simulink model "PV_model_final_02"  (R2021b)
settings: Solver=FixedStepDiscrete  StartTime=0.0  StopTime=80  FixedStep=Ts_Power  RelTol=1e-3
InitFcn:
  | freq = 60;
  | n = 100;
  | a = 20;
  | b = 10;
  | c = 150;
  | 
  | Fc = n * freq; % Carrier frequency, used for generating inverter SPWM signal (Hz)
  | Ts_Power = 1/(a * Fc); % SPS sample time (sec)
  | Ts_Control = b * Ts_Power; % Inverter control sample time (sec)
  | Ts_Data = c * Ts_Power; % Data storage and scope sample time (sec)
  | 
  | Dbias = 0.0;
  | Dupperlim = 0.5;
  | Dlowerlim = 0.2;
  | 
  | Ron=75e-3;
StopFcn:
  | %load('temp1.mat')
  | %[c,hist,edges,rmm,idx] = rainflow(temp.Data(:,3),temp.Time);
  | %histogram('BinEdges',edges','BinCounts',sum(hist,2));
  | %title('Histogram of S5 Thermal Cycles')
  | %xlabel('Temperature Cycle Range')
  | %ylabel('Cycle count')
undefined symbols (not defined in the file or in its folder): DiscIntNeverNeededParam
libraries: spsParallelRLCBranchLib x11, spsSeriesRLCBranchLib x6, spsMeanLib x6, spsIGBTDiodeLib x4, spsTHDLib x4, spsVoltageMeasurementLib x3, spsCurrentMeasurementLib x2, spsDiodeLib x2, spsGroundLib x2, slpidlib x2, spsControlledCurrentSourceLib x2, spsACVoltageSourceLib x1
settings Model: SimulationMode=accelerator  Creator=niall  LastModifiedBy=niall
settings DataIOCC: SaveOutput=off  DSMLogging=off  SaveTime=off  ReturnWorkspaceOutputs=off  SignalLoggingName=simout  LoggingToFile=on  LoggingFileName=simout.mat
settings DebuggingCC: ReadBeforeWriteMsg=DisableAll  WriteAfterWriteMsg=DisableAll  WriteAfterReadMsg=DisableAll  MultiTaskDSMMsg=none
settings ModelReferenceCC: UpdateModelReferenceTargets=IfOutOfDate
settings SFSimCC: SFSimEcho=off

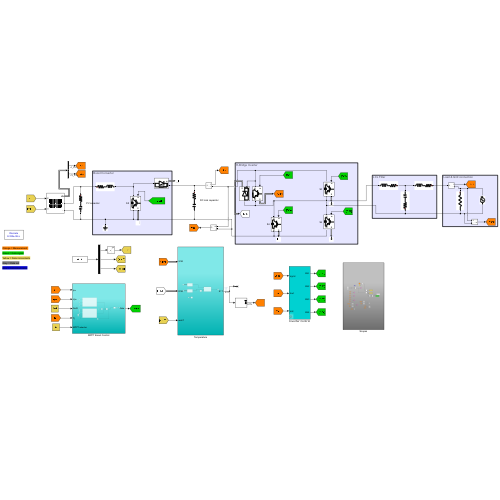
[thumbnail: Simulink's stored preview of the top-level diagram]
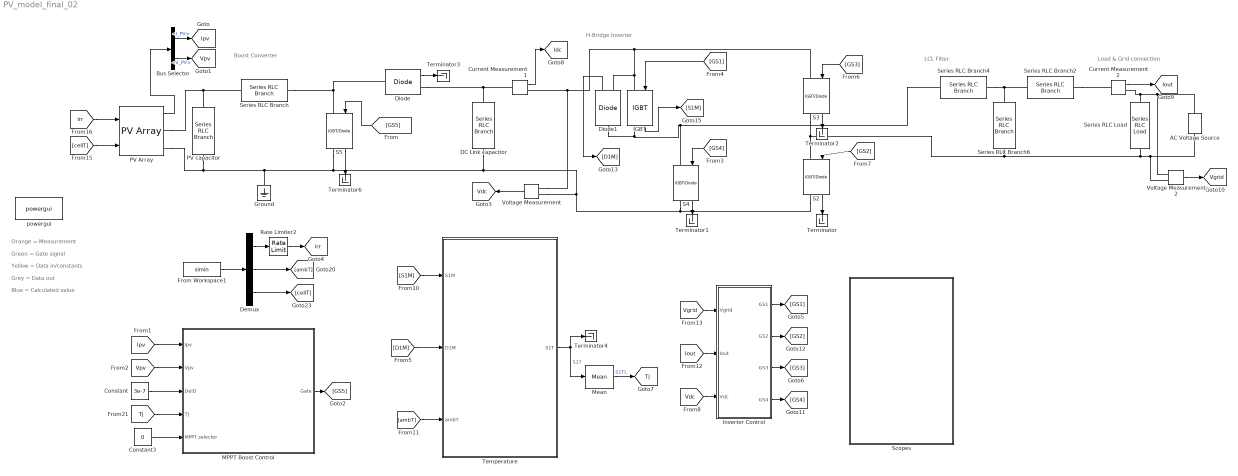
== system PV_model_final_02 ==
  note: Blue = Calculated value
  note: Grey = Data out
  note: Boost Converter
  note: H-Bridge Inverter
  note: LCL Filter
  note: Yellow = Data in/constants
  note: Green = Gate signal
  note: Orange = Measurement
  note: Load & Grid connection
  AC Voltage Source : spsACVoltageSourceLib/AC Voltage Source  Amplitude=240*sqrt(2)  Phase=0  Frequency=60  SampleTime=Ts_Power  Measurements=None  BusType=swing  Pref=10e3  Qref=0  Qmin=-inf  Qmax=+inf
  Bus Selector : BusSelector  OutputSignals=I_PV,V_PV
  Constant : Constant  Value=3e-7
  Constant3 : Constant  Value=0
  Current Measurement1 : spsCurrentMeasurementLib/Current Measurement  PhasorSimulation=off  OutputType=Complex  PSBequivalent=0
  Current Measurement2 : spsCurrentMeasurementLib/Current Measurement  PhasorSimulation=off  OutputType=Complex  PSBequivalent=0
  DC Link capacitor : spsSeriesRLCBranchLib/Series RLC Branch  LConnTagsString=__new0  RConnTagsString=__new0  BranchType=RC  Resistance=2.2e-3  Inductance=1e-3  SetiL0=off  InitialCurrent=0  Capacitance=2100e-6  Setx0=on  InitialVoltage=450  Measurements=None
  Demux : Demux  Outputs=3
  Diode : spsDiodeLib/Diode  Ron=0.001  Lon=0  Vf=0.8  IC=0  UseSnubber=0  Rs=500  Cs=250e-9  Measurements=on
  Diode1 : spsDiodeLib/Diode  Ron=10e-3  Lon=0  Vf=0.8  IC=0  UseSnubber=0  Rs=500  Cs=250e-9  Measurements=on
  From Workspace1 : FromWorkspace  VariableName=simin  SampleTime=Ts_Power  OutputAfterFinalValue=Holding final value
  Ground : spsGroundLib/Ground  LConnTagsString=a
  IGBT : spsIGBTLib/IGBT  Ron=Ron  Lon=0  Vf=2.2  Tf=1e-6  Tt=2e-6  IC=0  Rs=1e5  Cs=inf  Measurements=on
  Inverter Control : Subsystem  mask(Inverter Control){Pnom=10000, Fnom=60, Vnom_prim=240, Vnom_dc=450, Kp_VDCreg=10, Ki_VDCreg=50, Kp_Ireg=0.3, Ki_Ireg=9, RLff=[ 0.004 0.2 ], Fc=Fc, PWMmode12=Bipolar, Ts_Control=Ts_Control, Ts_PWMgenerator=Ts_Power}
      mask prompts: Pnom "Power (VA)"; Fnom "Frequency (Hz)"; Vnom_prim "Primary voltage (Vrms LL)"; Vnom_dc "DC voltage (V)"; Kp_VDCreg "Proportional gain"; Ki_VDCreg "Integral gain"; Kp_Ireg "Proportional gain"; Ki_Ireg "Integral gain"; RLff "Feedforward Values [Rff Lff] (pu)"; Fc "Carrier frequency (Hz)"; PWMmode12 "PWM method"; Ts_Control "Control systems"; Ts_PWMgenerator "PWM generator"
      mask help:
      | The main components of the Inverter Control are:
      | 1. PLL & Measurements
      | 2. Maximum Power Point Tracker System (MPPT) using a Perturb & Observe algorithm
      | 3. DC Voltage Regulator
      | 4. Current Regulator
      | 5. PWM Modulator
      mask init:
      | blockName=gcb;
      | if PWMmode12==1
      |     set_param([blockName,'/','PWM_Generator'],'ModulatorType','Single-phase full-bridge (4 pulses)')
      | else
      |     set_param([blockName,'/','PWM_Generator'],'ModulatorType','Single-phase full-bridge - Bipolar modulation (4 pulses)')
      | end
      mask TypeOptions PWMmode12: Unipolar | Bipolar
      mask DialogControl Container4 Prompt: Nominal Values:
      mask DialogControl Container8 Prompt: Dc Voltage Regulator:
      mask DialogControl Container6 Prompt: Current Regulator:
      mask DialogControl Container9 Prompt: PWM Modulator:
      mask DialogControl SampleTimes Prompt: Sample Times:
  MPPT Boost Control : Subsystem
  Mean : spsMeanLib/Mean  Freq=1  Vinit=20  Ts=Ts_Power
  PV Array : spsPVArrayLib/PV Array  Npar=2  Nser=9  PlotType=array @ 1000 W/m2 & specified temperatures  S_vec="[ 1000  500  100 ]"  Temp_C_vec="[ 45 25  ]"  ModuleName=User-defined  PlotWhenSelected=off  Pm=554.91  Ncell=110  Voc=38.1  Isc=18.56  Vm=31.8  Im=17.45  beta_Voc_pc=-0.25  alpha_Isc_pc=0.04  beta_Voc=-0.09525  alpha_Isc=0.007424  IL=18.6423  I0=6.4129e-12  nI=0.4702  Rsh=76.5819  Rs=0.11972  RobustModel=off  RobustCellTemperature=313.3991  BAL=on  Tc=1e-6  Tfilter=5e-5
  PV capacitor : spsSeriesRLCBranchLib/Series RLC Branch  LConnTagsString=__new0  RConnTagsString=__new0  BranchType=RC  Resistance=2.2e-3  Inductance=1e-3  SetiL0=off  InitialCurrent=0  Capacitance=2100e-6  Setx0=off  InitialVoltage=0  Measurements=None
  Rate Limiter2 : RateLimiter  RisingSlewLimit=2000  FallingSlewLimit=-2000  SampleTimeMode=inherited
  S{2..5} (4 alike) : spsIGBTDiodeLib/IGBT//Diode  Ron=Ron  Rs=1e5  Cs=inf  Measurements=on
  Scopes : Subsystem
  Series RLC Branch : spsSeriesRLCBranchLib/Series RLC Branch  LConnTagsString=__new0  RConnTagsString=__new0  BranchType=RL  Resistance=2e-3  Inductance=1.5e-3  SetiL0=off  InitialCurrent=0  Capacitance=1e-6  Setx0=off  InitialVoltage=0  Measurements=None
  Series RLC Branch2 : spsSeriesRLCBranchLib/Series RLC Branch  LConnTagsString=__new0  RConnTagsString=__new0  BranchType=RL  Resistance=4e-3  Inductance=4e-3  SetiL0=off  InitialCurrent=0  Capacitance=1e-6  Setx0=off  InitialVoltage=0  Measurements=None
  Series RLC Branch4 : spsSeriesRLCBranchLib/Series RLC Branch  LConnTagsString=__new0  RConnTagsString=__new0  BranchType=RL  Resistance=4e-3  Inductance=8e-3  SetiL0=off  InitialCurrent=0  Capacitance=1e-6  Setx0=off  InitialVoltage=0  Measurements=None
  Series RLC Branch6 : spsSeriesRLCBranchLib/Series RLC Branch  LConnTagsString=__new0  RConnTagsString=__new0  BranchType=RC  Resistance=2e-3  Inductance=1e-3  SetiL0=off  InitialCurrent=0  Capacitance=5e-6  Setx0=off  InitialVoltage=0  Measurements=None
  Series RLC Load : spsSeriesRLCLoadLib/Series RLC Load  LConnTagsString=a  RConnTagsString=__new0  NominalVoltage=240  NominalFrequency=60  ActivePower=10e3  InductivePower=0  CapacitivePower=0  Setx0=off  InitialVoltage=0  SetiL0=off  InitialCurrent=0  Measurements=None  LoadType=constant Z
  Temperature : Subsystem
  Terminator{,1..4,6} (6 alike) : Terminator
  Voltage Measurement : spsVoltageMeasurementLib/Voltage Measurement  PhasorSimulation=off  OutputType=Complex  PSBequivalent=0
  Voltage Measurement2 : spsVoltageMeasurementLib/Voltage Measurement  PhasorSimulation=off  OutputType=Complex  PSBequivalent=0
  powergui : spspowerguiLib/powergui  Priority=1  SimulationMode=Discrete  SampleTime=Ts_Power  frequency=60  Iterations=50  frequencyindice=0  Pbase=100e6  ErrMax=1e-4  UnitsV=kV  UnitsW=MW  buscounter=0  FunctionMessages=off  echomessages=off  EnableUseOfTLC=off  CurrentSourceSwitches=off  DisableSnubberDevices=off  DisableRonSwitches=off  DisableVfSwitches=off  DisplayEquations=off  AutomaticDiscreteSolvers=off  SolverType=Tustin/Backward Euler (TBE)  Interpol=off  ExternalGateDelay=off  methode=off  Ts=100  x0status=blocks  SPID=on  SwTol=0  HookPort=off  NonlinearTolerance=1e-4  nMaxIteration=100  ContinueOnMaxIteration=off  RestoreLinks=warning  ResistiveCurrentMeasurement=off  Frange=[0:2:500]  Ylog=off  Xlog=on  ShowGrid=off  save=off  variable=ZData  structure=0  ZoomFFT=off  StartTime=0.0  cycles=1  DisplayStyle=1  fundamental=60  FreqAxis=off  MaxFrequency=1000  frequencyindicesteady=1  RmsSteady=1  display=off
  tag scope: Idc=global, Iout=global, Ipv=global, Tj=global, Vdc=global, Vgrid=global, Vpv=global, irr=global
  wires:
  MPPT Boost Control/1(Gate) -> [GS5]
  [GS5] -> S5/1
  Current Measurement1/1 -> [Idc]
  [cellT] -> PV Array/2
  Bus Selector/2 -> [Vpv]  "<V_PV>"
  Voltage Measurement/1 -> [Vdc]
  Bus Selector/1 -> [Ipv]  "<I_PV>"
  [Ipv] -> MPPT Boost Control/1(Ipv)
  [Vpv] -> MPPT Boost Control/2(Vpv)
  Constant/1 -> MPPT Boost Control/3(DelD)
  PV Array/1 -> Bus Selector/1
  Current Measurement2/1 -> [Iout]
  Voltage Measurement2/1 -> [Vgrid]
  [Vdc] -> Inverter Control/3(Vdc)
  [Iout] -> Inverter Control/2(Iout)
  [Vgrid] -> Inverter Control/1(Vgrid)
  [GS1] -> IGBT/1
  [GS3] -> S3/1
  [GS4] -> S4/1
  [GS2] -> S2/1
  IGBT/1 -> [S1M]
  [S1M] -> Temperature/1(S1M)
  [ambT] -> Temperature/3(ambT)
  Inverter Control/1(GS1) -> [GS1]
  Inverter Control/2(GS2) -> [GS2]
  Inverter Control/3(GS3) -> [GS3]
  Inverter Control/4(GS4) -> [GS4]
  Temperature/1(S1T) -> Terminator4/1, Mean/1  "S1T"
  [Tj] -> MPPT Boost Control/4(Tj)
  Constant3/1 -> MPPT Boost Control/5(MPPT selector)
  Demux/1 -> Rate Limiter2/1
  From Workspace1/1 -> Demux/1
  Demux/2 -> [ambT]
  Demux/3 -> [cellT]
  S2/1 -> Terminator/1
  S4/1 -> Terminator1/1
  S3/1 -> Terminator2/1
  Diode/1 -> Terminator3/1
  Mean/1 -> [Tj]  "S1TL"
  [irr] -> PV Array/1
  Rate Limiter2/1 -> [irr]
  S5/1 -> Terminator6/1
  Diode1/1 -> [D1M]
  [D1M] -> Temperature/2(D1M)
  connections:
  DC Link capacitor/LConn1 -- Diode/RConn1 -- Current Measurement1/LConn1
  DC Link capacitor/RConn1 -- S5/RConn1 -- PV Array/RConn2 -- PV capacitor/RConn1 -- Ground/LConn1 -- S2/RConn1 -- S4/RConn1 -- Voltage Measurement/LConn2
  PV Array/RConn1 -- Series RLC Branch/LConn1 -- PV capacitor/LConn1
  S4/LConn1 -- Diode1/LConn1 -- IGBT/RConn1 -- Series RLC Branch4/RConn1
  AC Voltage Source/RConn1 -- Current Measurement2/RConn1 -- Series RLC Load/LConn1 -- Voltage Measurement2/LConn1
  Series RLC Branch4/LConn1 -- Series RLC Branch6/RConn1 -- Series RLC Branch2/RConn1
  Series RLC Branch/RConn1 -- S5/LConn1 -- Diode/LConn1
  Series RLC Load/RConn1 -- AC Voltage Source/LConn1 -- Voltage Measurement2/LConn2 -- S3/RConn1 -- S2/LConn1 -- Series RLC Branch6/LConn1
  Series RLC Branch2/LConn1 -- Current Measurement2/LConn1
  Voltage Measurement/LConn1 -- S3/LConn1 -- Diode1/RConn1 -- IGBT/LConn1 -- Current Measurement1/RConn1

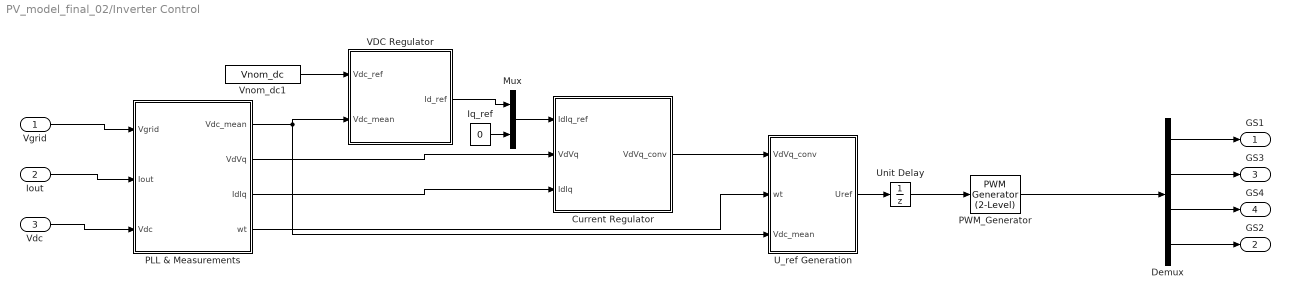
== system PV_model_final_02/Inverter Control ==
  Vgrid : Inport  PortDimensions=1
  Iout : Inport  Port=2  PortDimensions=1
  Vdc : Inport  Port=3  PortDimensions=1
  Current Regulator : Subsystem
  Demux : Demux
  Iq_ref : Constant  Value=0  SampleTime=Ts_Control
  Mux : Mux  Inputs=2
  PLL & Measurements : Subsystem
  PWM_Generator : spsPWMGenerator2LevelLib/PWM Generator (2-Level)  ModulatorType=Single-phase full-bridge - Bipolar modulation (4 pulses)  ModulatorMode=Unsynchronized  Fc=Fc  Pc=90  nF=27  MinMax="[ -1  1 ]"  SamplingTechnique=Asymmetrical regular (double edge)  ModulatingSignals=off  m=0.8  Freq=60  Phase=0  Ts=Ts_PWMgenerator  ShowCarrierOutport=off
      settings: AttributesFormatString=%<ModulatorType>
  "U_ref Generation " : Subsystem
  Unit Delay : UnitDelay  SampleTime=Ts_Control  HasFrameUpgradeWarning=on
  VDC Regulator : Subsystem
  Vnom_dc1 : Constant  Value=Vnom_dc  SampleTime=Ts_Control
  GS1 : Outport  VectorParamsAs1DForOutWhenUnconnected=off
  GS2 : Outport  Port=2  VectorParamsAs1DForOutWhenUnconnected=off
  GS3 : Outport  Port=3  VectorParamsAs1DForOutWhenUnconnected=off
  GS4 : Outport  Port=4  VectorParamsAs1DForOutWhenUnconnected=off
  wires:
  Iq_ref/1 -> Mux/2
  Vgrid/1 -> PLL & Measurements/1(Vgrid)
  Iout/1 -> PLL & Measurements/2(Iout)
  Unit Delay/1 -> PWM_Generator/1
  Vdc/1 -> PLL & Measurements/3(Vdc)
  PLL & Measurements/2(VdVq) -> Current Regulator/2(VdVq)
  PLL & Measurements/3(IdIq) -> Current Regulator/3(IdIq)
  Mux/1 -> Current Regulator/1(IdIq_ref)
  VDC Regulator/1(Id_ref) -> Mux/1
  PLL & Measurements/1(Vdc_mean) -> VDC Regulator/2(Vdc_mean), "U_ref Generation "/3(Vdc_mean)
  Current Regulator/1(VdVq_conv) -> "U_ref Generation "/1(VdVq_conv)
  PLL & Measurements/4(wt) -> "U_ref Generation "/2(wt)
  "U_ref Generation "/1(Uref) -> Unit Delay/1
  PWM_Generator/1 -> Demux/1
  Vnom_dc1/1 -> VDC Regulator/1(Vdc_ref)
  Demux/1 -> GS1/1
  Demux/2 -> GS3/1
  Demux/3 -> GS4/1
  Demux/4 -> GS2/1

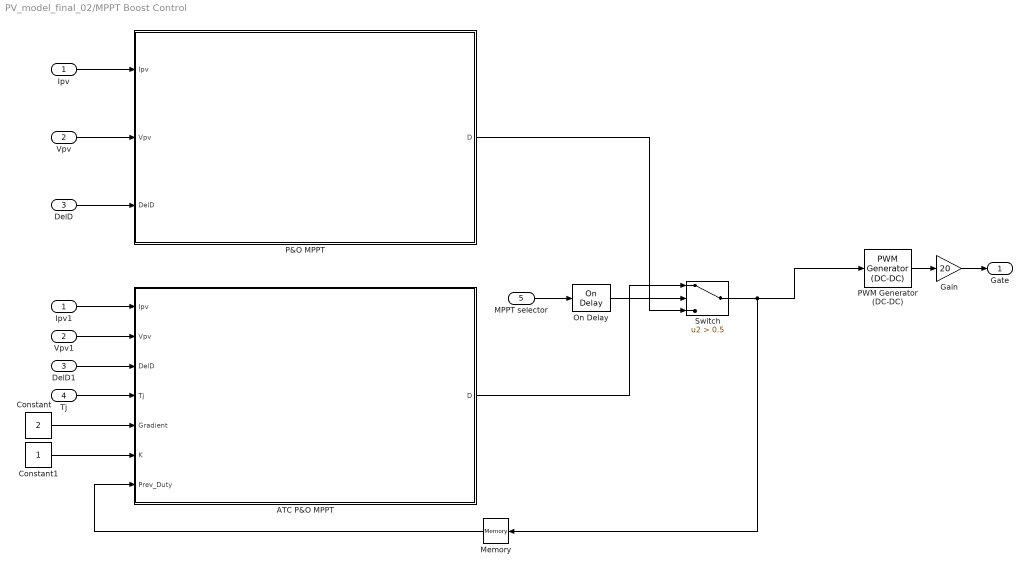
== system PV_model_final_02/MPPT Boost Control ==
  Ipv : Inport
  Vpv : Inport  Port=2
  DelD : Inport  Port=3
  Tj : Inport  Port=4
  MPPT selector : Inport  Port=5
  ATC P&O MPPT : Subsystem
  Constant : Constant  Value=2
  Constant1 : Constant
  DelD1 : InportShadow  Port=3
  Gain : Gain  Gain=20
  Ipv1 : InportShadow
  Memory : Memory
  On Delay : spsOnDelayLib/On Delay  DelayType=On delay  delay=5  ic=0  Ts=Ts_Control
      settings: SourceProductBaseCode=PS
  P&O MPPT : Subsystem
  PWM Generator (DC-DC) : spsPWMGeneratorDCDCLib/PWM Generator (DC-DC)  Fsw=5000  Ts=Ts_Power
  Switch : Switch  Criteria=u2 > Threshold  Threshold=0.5
  Vpv1 : InportShadow  Port=2
  Gate : Outport
  wires:
  Vpv/1 -> P&O MPPT/2(Vpv)
  Tj/1 -> ATC P&O MPPT/4(Tj)
  DelD/1 -> P&O MPPT/3(DelD)
  Ipv/1 -> P&O MPPT/1(Ipv)
  P&O MPPT/1(D) -> Switch/3
  DelD1/1 -> ATC P&O MPPT/3(DelD)
  Vpv1/1 -> ATC P&O MPPT/2(Vpv)
  Ipv1/1 -> ATC P&O MPPT/1(Ipv)
  ATC P&O MPPT/1(D) -> Switch/1
  MPPT selector/1 -> On Delay/1
  Constant/1 -> ATC P&O MPPT/5(Gradient)
  PWM Generator (DC-DC)/1 -> Gain/1
  Gain/1 -> Gate/1
  On Delay/1 -> Switch/2
  Memory/1 -> ATC P&O MPPT/7(Prev_Duty)
  Switch/1 -> PWM Generator (DC-DC)/1, Memory/1
  Constant1/1 -> ATC P&O MPPT/6(K)

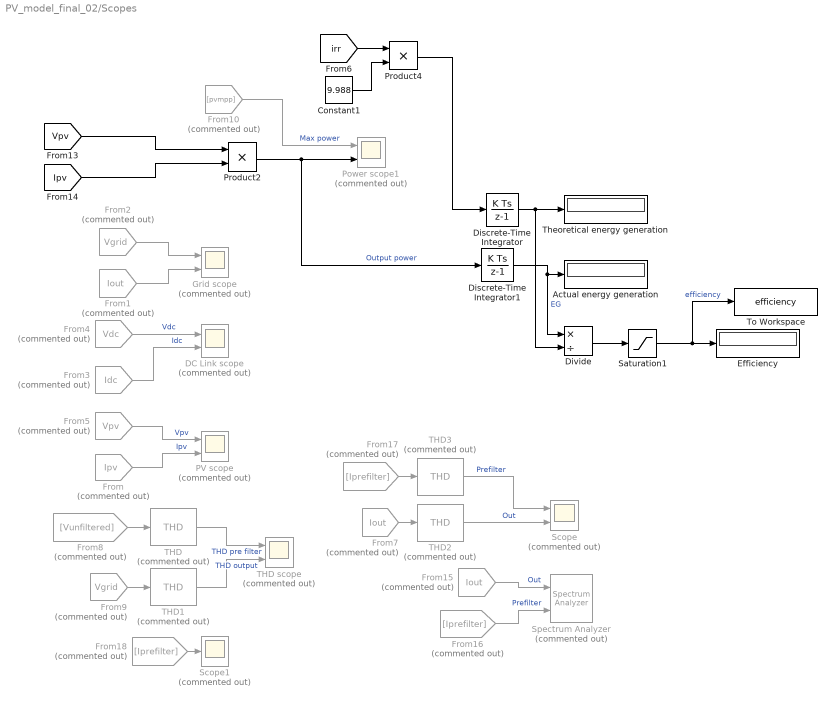
== system PV_model_final_02/Scopes ==
  Actual energy generation : Display
  Constant1 : Constant  Value=9.988  SampleTime=Ts_Power
  DC Link scope : Scope  Commented=on  NumInputPorts=2
  Discrete-Time Integrator : DiscreteIntegrator  SampleTime=Ts_Power  ICPrevOutput=DiscIntNeverNeededParam  ICPrevScaledInput=DiscIntNeverNeededParam
  Discrete-Time Integrator1 : DiscreteIntegrator  SampleTime=Ts_Power  ICPrevOutput=DiscIntNeverNeededParam  ICPrevScaledInput=DiscIntNeverNeededParam
  Divide : Product  Inputs=*/
  Efficiency : Display
  From : From  Commented=on  GotoTag=Ipv  TagVisibility=global
  From1 : From  Commented=on  GotoTag=Iout  TagVisibility=global
  From10 : From  Commented=on  GotoTag=pvmpp  TagVisibility=global
  From15 : From  Commented=on  GotoTag=Iout  TagVisibility=global
  From16 : From  Commented=on  GotoTag=Iprefilter  TagVisibility=global
  From17 : From  Commented=on  GotoTag=Iprefilter  TagVisibility=global
  From18 : From  Commented=on  GotoTag=Iprefilter  TagVisibility=global
  From2 : From  Commented=on  GotoTag=Vgrid  TagVisibility=global
  From3 : From  Commented=on  GotoTag=Idc  TagVisibility=global
  From4 : From  Commented=on  GotoTag=Vdc  TagVisibility=global
  From5 : From  Commented=on  GotoTag=Vpv  TagVisibility=global
  From7 : From  Commented=on  GotoTag=Iout  TagVisibility=global
  From8 : From  Commented=on  GotoTag=Vunfiltered
  From9 : From  Commented=on  GotoTag=Vgrid  TagVisibility=global
  Grid scope : Scope  Commented=on  NumInputPorts=2
  PV scope : Scope  Commented=on  NumInputPorts=2
  Power scope1 : Scope  Commented=on  NumInputPorts=2
  Product2 : Product
  Product4 : Product
  Saturation1 : Saturate  UpperLimit=1  LowerLimit=0
  Scope : Scope  Commented=on  NumInputPorts=2
  Scope1 : Scope  Commented=on
  Spectrum Analyzer : SpectrumAnalyzer  Commented=on  NumInputPorts=2
  THD{,1..3} (4 alike) : spsTHDLib/THD  Commented=on  Freq=60  Ts=Ts_Power
      settings: SourceProductBaseCode=PS
  THD scope : Scope  Commented=on  NumInputPorts=2
  Theoretical energy generation : Display
  To Workspace : ToWorkspace  VariableName=efficiency  SampleTime=60
      settings: MaxDataPoints=1
  wires:
  From3/1 -> DC Link scope/2  "Idc"
  From4/1 -> DC Link scope/1  "Vdc"
  [irr] -> Product4/1
  Constant1/1 -> Product4/2
  From/1 -> PV scope/2  "Ipv"
  From5/1 -> PV scope/1  "Vpv"
  THD/1 -> THD scope/1  "THD pre filter"
  THD1/1 -> THD scope/2  "THD output"
  From8/1 -> THD/1
  From9/1 -> THD1/1
  Discrete-Time Integrator/1 -> Divide/2, Theoretical energy generation/1
  Discrete-Time Integrator1/1 -> Divide/1, Actual energy generation/1  "EG"
  Divide/1 -> Saturation1/1
  Product4/1 -> Discrete-Time Integrator/1
  From10/1 -> Power scope1/1  "Max power"
  Product2/1 -> Discrete-Time Integrator1/1, Power scope1/2  "Output power"
  [Vpv] -> Product2/1
  From1/1 -> Grid scope/2
  From2/1 -> Grid scope/1
  THD2/1 -> Scope/2  "Out"
  From7/1 -> THD2/1
  From15/1 -> Spectrum Analyzer/1  "Out"
  From16/1 -> Spectrum Analyzer/2  "Prefilter"
  From17/1 -> THD3/1
  THD3/1 -> Scope/1  "Prefilter"
  From18/1 -> Scope1/1
  Saturation1/1 -> To Workspace/1, Efficiency/1  "efficiency"
  [Ipv] -> Product2/2

== system PV_model_final_02/Temperature ==
  S1M : Inport
  D1M : Inport  Port=2
  ambT : Inport  Port=3
  Diode losses : Subsystem
  IGBT losses : Subsystem
  Thermal Model : Subsystem
  S1T : Outport
  wires:
  IGBT losses/1(PLoss) -> Thermal Model/1(IGBT Power Loss)  "IGBT"
  Diode losses/1(PLoss) -> Thermal Model/2(Diode Power Loss)  "DIODE"
  S1M/1 -> IGBT losses/1(m)
  Thermal Model/1(Tj) -> S1T/1  "S1T"
  ambT/1 -> [AmbT]
  [AmbT] -> Thermal Model/3(Ambient T)
  D1M/1 -> Diode losses/1(m)

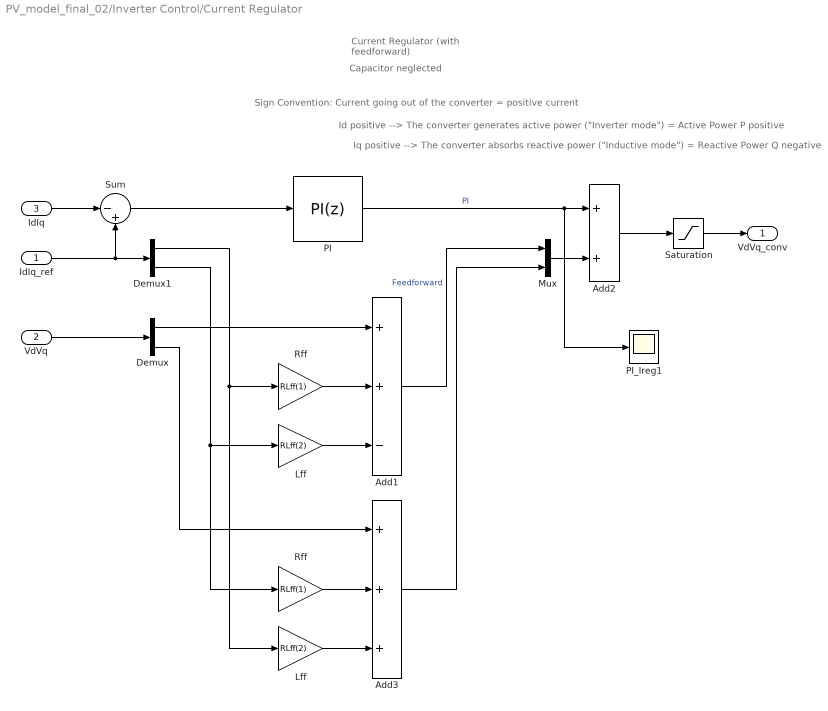
== system PV_model_final_02/Inverter Control/Current Regulator ==
  note: Id positive --> The converter generates active power ("Inverter mode") = Active Power P positive
  note: Iq positive --> The converter absorbs reactive power ("Inductive mode") = Reactive Power Q negative
  note: Sign Convention: Current going out of the converter = positive current
  note: Current Regulator
      | (with feedforward)
  note: Capacitor neglected
  IdIq_ref : Inport  PortDimensions=2
  VdVq : Inport  Port=2  PortDimensions=2
  IdIq : Inport  Port=3  PortDimensions=2
  Add1 : Sum  Inputs=++-
  Add2 : Sum
  Add3 : Sum  Inputs=+++
  Demux : Demux  Outputs=2
  Demux1 : Demux  Outputs=2
  Lff : Gain  Gain=RLff(2)  SaturateOnIntegerOverflow=on  OutDataTypeStr=Inherit: Same as input  ParamDataTypeStr=Inherit: Same as input
  "Lff  " : Gain  Gain=RLff(2)  SaturateOnIntegerOverflow=on  OutDataTypeStr=Inherit: Same as input  ParamDataTypeStr=Inherit: Same as input
  Mux : Mux  Inputs=2
  PI : slpidlib/PID Controller  Controller=PI  Form=Parallel  TimeDomain=Discrete-time  UseExternalTs=off  SampleTime=Ts_Control  IntegratorMethod=Forward Euler  FilterMethod=Forward Euler  ControllerParametersSource=internal  P=Kp_Ireg  I=Ki_Ireg  D=0  UseFilter=on  N=100  TunerSelectOption=Transfer Function Based (PID Tuner App)  InitialConditionSource=internal  InitialConditionForIntegrator=0  InitialConditionForFilter=0  DifferentiatorICPrevScaledInput=0  ExternalReset=none  TrackingMode=off  Kt=1  LimitOutput=on  SatLimitsSource=internal  UpperSaturationLimit=2  LowerSaturationLimit=-2  LinearizeAsGain=off  AntiWindupMode=none  Kb=1  POutMin=[]  POutMax=[]  IOutMin=[]  IOutMax=[]  DOutMin=[]  DOutMax=[]  NOutMin=[]  NOutMax=[]  SumOutMin=[]  SumOutMax=[]  SaturationOutMin=[]  SaturationOutMax=[]  PParamMin=[]  PParamMax=[]  IParamMin=[]  IParamMax=[]  DParamMin=[]  DParamMax=[]  NParamMin=[]  NParamMax=[]  KbParamMin=[]  KbParamMax=[]  KtParamMin=[]  KtParamMax=[]  KbOutMin=[]  KbOutMax=[]  KtOutMin=[]  KtOutMax=[]  IntegratorOutMin=[]  IntegratorOutMax=[]  FilterOutMin=[]  FilterOutMax=[]  SumI1OutMin=[]  SumI1OutMax=[]  SumI2OutMin=[]  SumI2OutMax=[]  SumI3OutMin=[]  SumI3OutMax=[]  SumI4OutMin=[]  SumI4OutMax=[]  SumDOutMin=[]  SumDOutMax=[]  DifferentiatorOutMin=[]  DifferentiatorOutMax=[]  FilterDiffOutCoefMin=[]  FilterDiffOutCoefMax=[]  ReciprocalOutMin=[]  ReciprocalOutMax=[]  SumDenOutMin=[]  SumDenOutMax=[]  SumNumOutMin=[]  SumNumOutMax=[]  DivideOutMin=[]  DivideOutMax=[]  UdiffTsProdOutMin=[]  UdiffTsProdOutMax=[]  NTsProdOutMin=[]  NTsProdOutMax=[]  UintegralTsProdOutMin=[]  UintegralTsProdOutMax=[]  UngainTsProdOutMin=[]  UngainTsProdOutMax=[]  IntegratorContinuousStateAttributes=''  IntegratorStateMustResolveToSignalObject=off  IntegratorRTWStateStorageClass=Auto  FilterContinuousStateAttributes=''  FilterStateMustResolveToSignalObject=off  FilterRTWStateStorageClass=Auto  ParallelPVariant=InternalParameters  IdealPVariant=Disabled  IVariant=InternalParameters  DVariant=Disabled  IntegratorVariant=Discrete  SatVariant=Enabled  AWVariant=Passthrough  PCopyVariant=Disabled  TRVariant=Disabled  FdbkBlocksVariant=Forward  IdealPFdbkVariant=Disabled  SatFdbkVariant=Disabled  DerivativeFilterVariant=Disabled  NVariant=Disabled  NCopyVariant=Disabled_SignalSpec  FilterICVariant=Disabled  IntegratorICVariant=InternalICs  ExternalResetVariant=Disabled  TRSumVariant=Passthrough  SumFdbkVariant=Disabled  SumVariant=Sum_PI  TsampFilterVariant=InternalTs  TsampNgainVariant=Passthrough  TsampIntegralVariant=Passthrough  ExternalSaturationOutDataTypeStr=Inherit: Same as second input
  PI_Ireg1 : Scope
  Rff : Gain  Gain=RLff(1)  SaturateOnIntegerOverflow=on  OutDataTypeStr=Inherit: Same as input  ParamDataTypeStr=Inherit: Same as input
  "Rff " : Gain  Gain=RLff(1)  SaturateOnIntegerOverflow=on  OutDataTypeStr=Inherit: Same as input  ParamDataTypeStr=Inherit: Same as input
  Saturation : Saturate  UpperLimit=1.5  LowerLimit=-1.5
  Sum : Sum  Inputs=|-+
  VdVq_conv : Outport  VectorParamsAs1DForOutWhenUnconnected=off
  wires:
  Add3/1 -> Mux/2
  Demux/2 -> Add3/1
  Add1/1 -> Mux/1  "Feedforward"
  Lff/1 -> Add3/3
  Rff/1 -> Add3/2
  Demux1/2 -> Rff/1, "Lff  "/1
  "Lff  "/1 -> Add1/3
  Demux1/1 -> Lff/1, "Rff "/1
  "Rff "/1 -> Add1/2
  Demux/1 -> Add1/1
  VdVq/1 -> Demux/1
  Saturation/1 -> VdVq_conv/1
  Add2/1 -> Saturation/1
  IdIq/1 -> Sum/1
  IdIq_ref/1 -> Demux1/1, Sum/2
  Sum/1 -> PI/1
  PI/1 -> Add2/1, PI_Ireg1/1  "PI"
  Mux/1 -> Add2/2

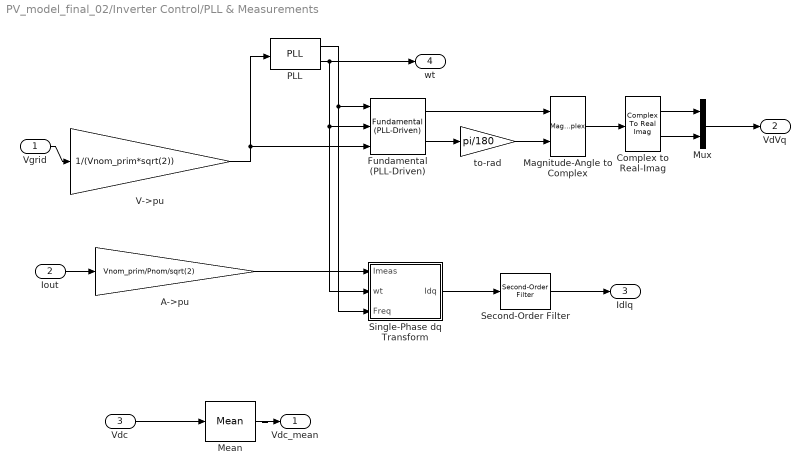
== system PV_model_final_02/Inverter Control/PLL & Measurements ==
  Vgrid : Inport
  Iout : Inport  Port=2
  Vdc : Inport  Port=3
  A->pu : Gain  Gain=Vnom_prim/Pnom/sqrt(2)  SaturateOnIntegerOverflow=on  OutDataTypeStr=Inherit: Same as input  ParamDataTypeStr=Inherit: Same as input
  Complex to Real-Imag : ComplexToRealImag
  Fundamental (PLL-Driven) : spsFundamentalPLLDrivenLib/Fundamental (PLL-Driven)  Finit=Fnom  Fmin=45  InInit=[1, 0]  Ts=Ts_Control
      settings: SourceProductBaseCode=PS
  Magnitude-Angle to Complex : MagnitudeAngleToComplex
  Mean : spsMeanLib/Mean  Freq=Fnom  Vinit=Vnom_dc  Ts=Ts_Control
  Mux : Mux  Inputs=2
  PLL : spsPLLLib/PLL  Fmin=45  Par_Init=[0, Fnom]  ParK=[180, 3200, 1]  TcD=1e-4  MaxRateChangeFreq=12  FilterCutOffFreq=25  Ts=Ts_Control  AGC=on
      settings: SourceProductBaseCode=PS
  Second-Order Filter : spsSecondOrderFilterLib/Second-Order Filter  FilterType=Lowpass  Fo=2000  Zeta=1  Ts=Ts_Control  Initialize=on  Vac_Init="[0,  0,  50;0,0,50]"  Vdc_Init=[0.9 0]  PlotResponse=off  FreqRange=[0, 500, 1]
      settings: SourceProductBaseCode=PS
  Single-Phase dq Transform : Subsystem
  V->pu : Gain  Gain=1/(Vnom_prim*sqrt(2))  SaturateOnIntegerOverflow=on  OutDataTypeStr=Inherit: Same as input  ParamDataTypeStr=Inherit: Same as input
  to-rad : Gain  Gain=pi/180
  Vdc_mean : Outport  VectorParamsAs1DForOutWhenUnconnected=off
  VdVq : Outport  Port=2  VectorParamsAs1DForOutWhenUnconnected=off
  IdIq : Outport  Port=3  VectorParamsAs1DForOutWhenUnconnected=off
  wt : Outport  Port=4  VectorParamsAs1DForOutWhenUnconnected=off
  wires:
  Mean/1 -> Vdc_mean/1
  Vdc/1 -> Mean/1
  to-rad/1 -> Magnitude-Angle to Complex/2
  Mux/1 -> VdVq/1
  Complex to Real-Imag/2 -> Mux/2
  Complex to Real-Imag/1 -> Mux/1
  Magnitude-Angle to Complex/1 -> Complex to Real-Imag/1
  Fundamental (PLL-Driven)/2 -> to-rad/1
  Fundamental (PLL-Driven)/1 -> Magnitude-Angle to Complex/1
  A->pu/1 -> Single-Phase dq Transform/1(Imeas)
  PLL/1 -> Single-Phase dq Transform/3(Freq), Fundamental (PLL-Driven)/1
  PLL/2 -> wt/1, Fundamental (PLL-Driven)/2, Single-Phase dq Transform/2(wt)
  Iout/1 -> A->pu/1
  Vgrid/1 -> V->pu/1
  V->pu/1 -> Fundamental (PLL-Driven)/3, PLL/1
  Single-Phase dq Transform/1(Idq) -> Second-Order Filter/1
  Second-Order Filter/1 -> IdIq/1

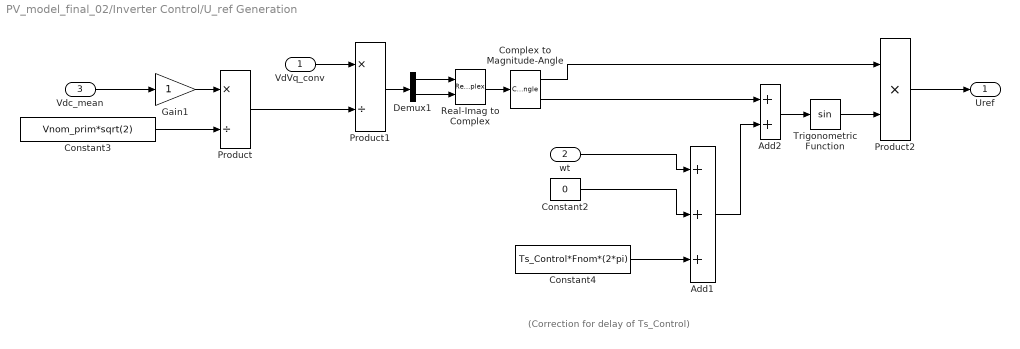
== system PV_model_final_02/Inverter Control/U_ref Generation  ==
  note: (Correction for delay of Ts_Control)
  VdVq_conv : Inport
  wt : Inport  Port=2
  Vdc_mean : Inport  Port=3
  Add1 : Sum  Inputs=+++
  Add2 : Sum
  Complex to Magnitude-Angle : ComplexToMagnitudeAngle
  Constant2 : Constant  Value=0  SampleTime=Ts_Control
  Constant3 : Constant  Value=Vnom_prim*sqrt(2)  SampleTime=Ts_Control
  Constant4 : Constant  Value=Ts_Control*Fnom*(2*pi)  SampleTime=Ts_Control
  Demux1 : Demux  Outputs=2
  Gain1 : Gain
  Product : Product  Inputs=*/  RndMeth=Zero
  Product1 : Product  Inputs=*/  RndMeth=Zero
  Product2 : Product  Inputs=**  RndMeth=Zero
  Real-Imag to Complex : RealImagToComplex
  Trigonometric Function : Trigonometry
  Uref : Outport  VectorParamsAs1DForOutWhenUnconnected=off
  wires:
  VdVq_conv/1 -> Product1/1
  Product2/1 -> Uref/1
  Constant4/1 -> Add1/3
  wt/1 -> Add1/1
  Trigonometric Function/1 -> Product2/2
  Complex to Magnitude-Angle/1 -> Product2/1
  Add2/1 -> Trigonometric Function/1
  Add1/1 -> Add2/2
  Complex to Magnitude-Angle/2 -> Add2/1
  Product/1 -> Product1/2
  Constant3/1 -> Product/2
  Constant2/1 -> Add1/2
  Demux1/2 -> Real-Imag to Complex/2
  Demux1/1 -> Real-Imag to Complex/1
  Real-Imag to Complex/1 -> Complex to Magnitude-Angle/1
  Gain1/1 -> Product/1
  Product1/1 -> Demux1/1
  Vdc_mean/1 -> Gain1/1

== system PV_model_final_02/Inverter Control/VDC Regulator ==
  Vdc_ref : Inport  PortDimensions=1
  Vdc_mean : Inport  Port=2  PortDimensions=1
  PI : slpidlib/PID Controller  Controller=PI  Form=Parallel  TimeDomain=Discrete-time  UseExternalTs=off  SampleTime=Ts_Control  IntegratorMethod=Trapezoidal  FilterMethod=Forward Euler  ControllerParametersSource=internal  P=Kp_VDCreg  I=Ki_VDCreg  D=0  UseFilter=on  N=100  TunerSelectOption=Transfer Function Based (PID Tuner App)  InitialConditionSource=internal  InitialConditionForIntegrator=0.9226  InitialConditionForFilter=0  DifferentiatorICPrevScaledInput=0  ExternalReset=none  TrackingMode=off  Kt=1  LimitOutput=on  SatLimitsSource=internal  UpperSaturationLimit=1.5  LowerSaturationLimit=-1.5  LinearizeAsGain=off  AntiWindupMode=none  Kb=1  POutMin=[]  POutMax=[]  IOutMin=[]  IOutMax=[]  DOutMin=[]  DOutMax=[]  NOutMin=[]  NOutMax=[]  SumOutMin=[]  SumOutMax=[]  SaturationOutMin=[]  SaturationOutMax=[]  PParamMin=[]  PParamMax=[]  IParamMin=[]  IParamMax=[]  DParamMin=[]  DParamMax=[]  NParamMin=[]  NParamMax=[]  KbParamMin=[]  KbParamMax=[]  KtParamMin=[]  KtParamMax=[]  KbOutMin=[]  KbOutMax=[]  KtOutMin=[]  KtOutMax=[]  IntegratorOutMin=[]  IntegratorOutMax=[]  FilterOutMin=[]  FilterOutMax=[]  SumI1OutMin=[]  SumI1OutMax=[]  SumI2OutMin=[]  SumI2OutMax=[]  SumI3OutMin=[]  SumI3OutMax=[]  SumI4OutMin=[]  SumI4OutMax=[]  SumDOutMin=[]  SumDOutMax=[]  DifferentiatorOutMin=[]  DifferentiatorOutMax=[]  FilterDiffOutCoefMin=[]  FilterDiffOutCoefMax=[]  ReciprocalOutMin=[]  ReciprocalOutMax=[]  SumDenOutMin=[]  SumDenOutMax=[]  SumNumOutMin=[]  SumNumOutMax=[]  DivideOutMin=[]  DivideOutMax=[]  UdiffTsProdOutMin=[]  UdiffTsProdOutMax=[]  NTsProdOutMin=[]  NTsProdOutMax=[]  UintegralTsProdOutMin=[]  UintegralTsProdOutMax=[]  UngainTsProdOutMin=[]  UngainTsProdOutMax=[]  IntegratorContinuousStateAttributes=''  IntegratorStateMustResolveToSignalObject=off  IntegratorRTWStateStorageClass=Auto  FilterContinuousStateAttributes=''  FilterStateMustResolveToSignalObject=off  FilterRTWStateStorageClass=Auto  ParallelPVariant=InternalParameters  IdealPVariant=Disabled  IVariant=InternalParameters  DVariant=Disabled  IntegratorVariant=Discrete  SatVariant=Enabled  AWVariant=Passthrough  PCopyVariant=Disabled  TRVariant=Disabled  FdbkBlocksVariant=Forward  IdealPFdbkVariant=Disabled  SatFdbkVariant=Disabled  DerivativeFilterVariant=Disabled  NVariant=Disabled  NCopyVariant=Disabled_SignalSpec  FilterICVariant=Disabled  IntegratorICVariant=InternalICs  ExternalResetVariant=Disabled  TRSumVariant=Passthrough  SumFdbkVariant=Disabled  SumVariant=Sum_PI  TsampFilterVariant=InternalTs  TsampNgainVariant=Passthrough  TsampIntegralVariant=Passthrough  ExternalSaturationOutDataTypeStr=Inherit: Same as second input
  Rtot_pu2 : Gain  Gain=1/Vnom_dc  SaturateOnIntegerOverflow=on  OutDataTypeStr=Inherit: Same as input  ParamDataTypeStr=Inherit: Same as input
  Sum : Sum  Inputs=|+-
  Id_ref : Outport  InitialOutput=0  VectorParamsAs1DForOutWhenUnconnected=off
  wires:
  Rtot_pu2/1 -> PI/1
  Vdc_ref/1 -> Sum/2
  Vdc_mean/1 -> Sum/1
  Sum/1 -> Rtot_pu2/1
  PI/1 -> Id_ref/1

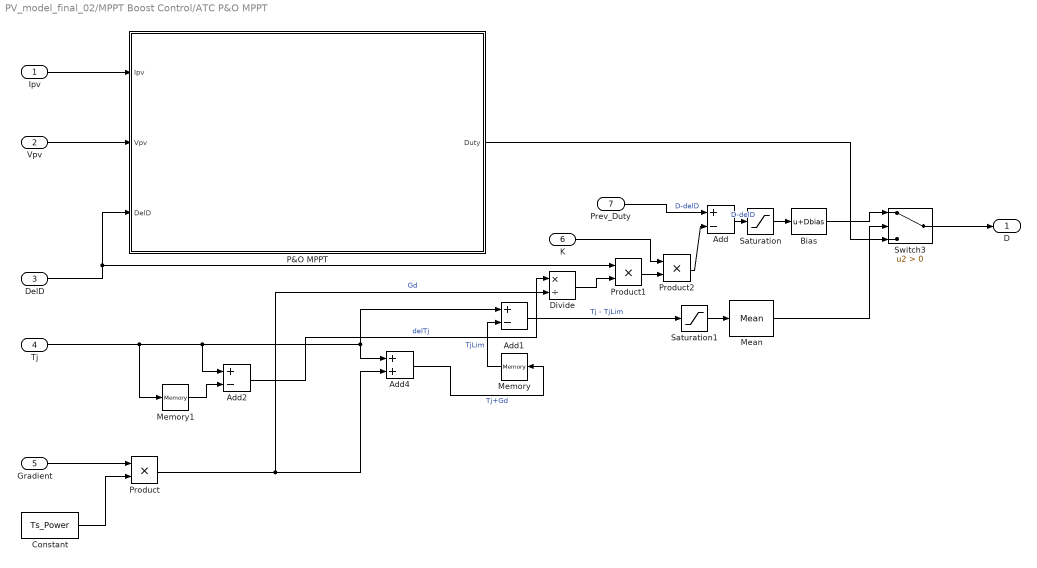
== system PV_model_final_02/MPPT Boost Control/ATC P&O MPPT ==
  Ipv : Inport
  Vpv : Inport  Port=2
  DelD : Inport  Port=3
  Tj : Inport  Port=4
  Gradient : Inport  Port=5
  K : Inport  Port=6
  Prev_Duty : Inport  Port=7
  Add : Sum  Inputs=+-
  Add1 : Sum  Inputs=+-
  Add2 : Sum  Inputs=+-
  Add4 : Sum
  Bias : Bias  Bias=Dbias
  Constant : Constant  Value=Ts_Power
  Divide : Product  Inputs=*/
  Mean : spsMeanLib/Mean  Freq=60  Vinit=0  Ts=Ts_Power
  Memory : Memory
  Memory1 : Memory
  P&O MPPT : Subsystem
  Product : Product
  Product1 : Product
  Product2 : Product
  Saturation : Saturate  UpperLimit=Dupperlim  LowerLimit=Dlowerlim
  Saturation1 : Saturate  UpperLimit=2e-3  LowerLimit=-2e-3
  Switch3 : Switch  Criteria=u2 > Threshold
  D : Outport
  wires:
  K/1 -> Product2/1
  Product2/1 -> Add/2
  Product1/1 -> Product2/2
  Add2/1 -> Divide/1  "delTj"
  Gradient/1 -> Product/1
  Mean/1 -> Switch3/2
  Switch3/1 -> D/1
  P&O MPPT/1(Duty) -> Switch3/3
  Ipv/1 -> P&O MPPT/1(Ipv)
  Vpv/1 -> P&O MPPT/2(Vpv)
  Saturation/1 -> Bias/1
  Saturation1/1 -> Mean/1
  Memory/1 -> Add1/2  "TjLim"
  Add/1 -> Saturation/1  "D-delD"
  Product/1 -> Divide/2, Add4/2  "Gd"
  Memory1/1 -> Add2/2
  Prev_Duty/1 -> Add/1  "D-delD"
  Add4/1 -> Memory/1  "Tj+Gd"
  Constant/1 -> Product/2
  Divide/1 -> Product1/2
  Tj/1 -> Add1/1, Add4/1, Add2/1, Memory1/1
  DelD/1 -> Product1/1, P&O MPPT/3(DelD)
  Add1/1 -> Saturation1/1  "Tj - TjLim"
  Bias/1 -> Switch3/1

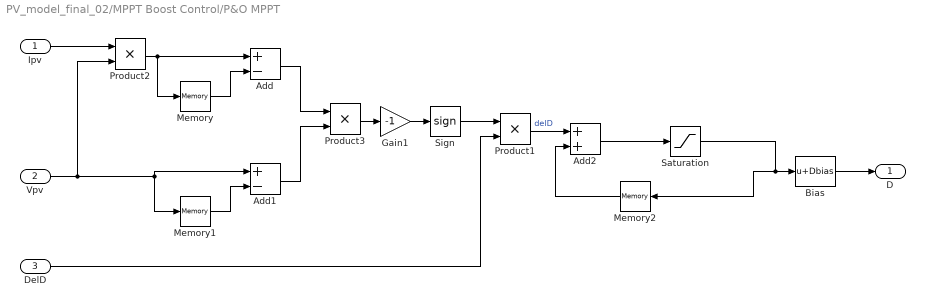
== system PV_model_final_02/MPPT Boost Control/P&O MPPT ==
  Ipv : Inport
  Vpv : Inport  Port=2
  DelD : Inport  Port=3
  Add : Sum  Inputs=+-
  Add1 : Sum  Inputs=+-
  Add2 : Sum
  Bias : Bias  Bias=Dbias
  Gain1 : Gain  Gain=-1
  Memory : Memory
  Memory1 : Memory
  Memory2 : Memory
  Product1 : Product
  Product2 : Product
  Product3 : Product
  Saturation : Saturate  UpperLimit=Dupperlim  LowerLimit=Dlowerlim
  Sign : Signum
  D : Outport
  wires:
  Product3/1 -> Gain1/1
  Product1/1 -> Add2/1  "delD"
  Ipv/1 -> Product2/1
  Sign/1 -> Product1/1
  Add/1 -> Product3/1
  Memory1/1 -> Add1/2
  Memory2/1 -> Add2/2
  Memory/1 -> Add/2
  Product2/1 -> Memory/1, Add/1
  Add1/1 -> Product3/2
  Gain1/1 -> Sign/1
  DelD/1 -> Product1/2
  Vpv/1 -> Add1/1, Memory1/1, Product2/2
  Saturation/1 -> Bias/1, Memory2/1
  Add2/1 -> Saturation/1
  Bias/1 -> D/1

== system PV_model_final_02/Temperature/Diode losses ==
  m : Inport
  Demux : Demux  Outputs=2
  Mean2 : spsMeanLib/Mean  Freq=Fc  Vinit=0  Ts=Ts_Power
  Product : Product
  Saturation : Saturate  UpperLimit=1000  LowerLimit=0.8
  PLoss : Outport
  wires:
  m/1 -> Demux/1
  Saturation/1 -> Product/2
  Product/1 -> Mean2/1
  Demux/2 -> Saturation/1
  Demux/1 -> Product/1
  Mean2/1 -> PLoss/1

== system PV_model_final_02/Temperature/IGBT losses ==
  m : Inport
  Add : Sum
  Add1 : Sum
  Constant1 : Constant  Value=0.325
  Constant2 : Constant  Value=Fc
  Demux : Demux  Outputs=2
  Eoff : Constant  Value=0.58e-3
  Eon : Constant  Value=1.1e-3
  Mean : spsMeanLib/Mean  Freq=Fc  Vinit=0  Ts=Ts_Power
  Product3 : Product  Inputs=3
  Product4 : Product
  Saturation : Saturate  UpperLimit=100  LowerLimit=0
  PLoss : Outport
  wires:
  m/1 -> Demux/1
  Add1/1 -> PLoss/1
  Demux/2 -> Product3/2
  Constant1/1 -> Product3/3
  Product3/1 -> Mean/1
  Demux/1 -> Saturation/1
  Constant2/1 -> Product4/2
  Add/1 -> Product4/1
  Eon/1 -> Add/1
  Eoff/1 -> Add/2
  Product4/1 -> Add1/2
  Mean/1 -> Add1/1
  Saturation/1 -> Product3/1

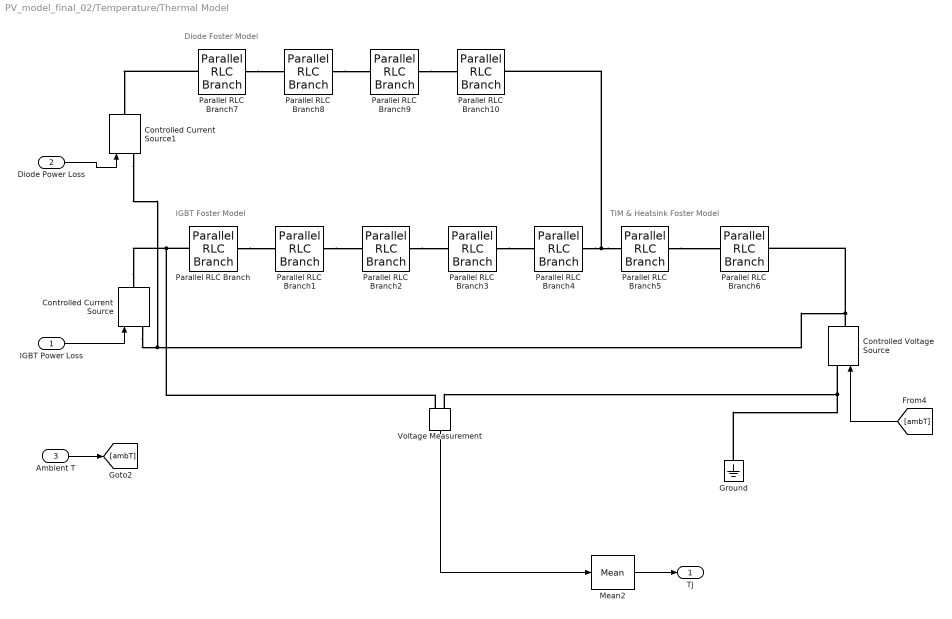
== system PV_model_final_02/Temperature/Thermal Model ==
  note: Diode Foster Model
  note: IGBT Foster Model
  note: TIM & Heatsink Foster Model
  IGBT Power Loss : Inport
  Diode Power Loss : Inport  Port=2
  Ambient T : Inport  Port=3
  Controlled Current Source : spsControlledCurrentSourceLib/Controlled Current Source  Initialize=on  Source_Type=DC  Amplitude=0  Phase=0  Frequency=0  Measurements=None
  Controlled Current Source1 : spsControlledCurrentSourceLib/Controlled Current Source  Initialize=on  Source_Type=DC  Amplitude=0  Phase=0  Frequency=0  Measurements=None
  Controlled Voltage Source : spsControlledVoltageSourceLib/Controlled Voltage Source  Initialize=on  Source_Type=DC  Amplitude=0  Phase=0  Frequency=0  Measurements=None
  Ground : spsGroundLib/Ground  LConnTagsString=a
  Mean2 : spsMeanLib/Mean  Freq=Fc/30  Vinit=0  Ts=Ts_Power
  Parallel RLC Branch : spsParallelRLCBranchLib/Parallel RLC Branch  LConnTagsString=a  RConnTagsString=__new0  BranchType=RC  Resistance=0.02540725  Inductance=1e-3  SetiL0=off  InitialCurrent=0  Capacitance=1.3e-5/0.02540725  Setx0=off  InitialVoltage=0  Measurements=None
  Parallel RLC Branch1 : spsParallelRLCBranchLib/Parallel RLC Branch  LConnTagsString=a  RConnTagsString=__new0  BranchType=RC  Resistance=0.09179841  Inductance=1e-3  SetiL0=off  InitialCurrent=0  Capacitance=1.3e-4/0.09179841  Setx0=off  InitialVoltage=0  Measurements=None
  Parallel RLC Branch10 : spsParallelRLCBranchLib/Parallel RLC Branch  LConnTagsString=a  RConnTagsString=__new0  BranchType=RC  Resistance=0.1348257  Inductance=1e-3  SetiL0=off  InitialCurrent=0  Capacitance=0.09207449/0.1348257  Setx0=off  InitialVoltage=0  Measurements=None
  Parallel RLC Branch2 : spsParallelRLCBranchLib/Parallel RLC Branch  LConnTagsString=a  RConnTagsString=__new0  BranchType=RC  Resistance=0.1302173  Inductance=1e-3  SetiL0=off  InitialCurrent=0  Capacitance=1.4e-3/0.1302173  Setx0=off  InitialVoltage=0  Measurements=None
  Parallel RLC Branch3 : spsParallelRLCBranchLib/Parallel RLC Branch  LConnTagsString=a  RConnTagsString=__new0  BranchType=RC  Resistance=0.1893012  Inductance=1e-3  SetiL0=off  InitialCurrent=0  Capacitance=0.01830399/0.1893012  Setx0=off  InitialVoltage=0  Measurements=None
  Parallel RLC Branch4 : spsParallelRLCBranchLib/Parallel RLC Branch  LConnTagsString=a  RConnTagsString=__new0  BranchType=RC  Resistance=0.0532358  Inductance=1e-3  SetiL0=off  InitialCurrent=0  Capacitance=0.1308578/0.0532358  Setx0=off  InitialVoltage=0  Measurements=None
  Parallel RLC Branch5 : spsParallelRLCBranchLib/Parallel RLC Branch  LConnTagsString=a  RConnTagsString=__new0  BranchType=R  Resistance=0.0005  Inductance=1e-3  SetiL0=off  InitialCurrent=0  Capacitance=1e-6  Setx0=off  InitialVoltage=0  Measurements=None
  Parallel RLC Branch6 : spsParallelRLCBranchLib/Parallel RLC Branch  LConnTagsString=a  RConnTagsString=__new0  BranchType=RC  Resistance=2  Inductance=1e-3  SetiL0=off  InitialCurrent=0  Capacitance=20/2  Setx0=off  InitialVoltage=0  Measurements=None
  Parallel RLC Branch7 : spsParallelRLCBranchLib/Parallel RLC Branch  LConnTagsString=a  RConnTagsString=__new0  BranchType=RC  Resistance=0.3399738  Inductance=1e-3  SetiL0=off  InitialCurrent=0  Capacitance=1.3e-4/0.3399738  Setx0=off  InitialVoltage=0  Measurements=None
  Parallel RLC Branch8 : spsParallelRLCBranchLib/Parallel RLC Branch  LConnTagsString=a  RConnTagsString=__new0  BranchType=RC  Resistance=0.4445632  Inductance=1e-3  SetiL0=off  InitialCurrent=0  Capacitance=1.5e-3/0.4445632  Setx0=off  InitialVoltage=0  Measurements=None
  Parallel RLC Branch9 : spsParallelRLCBranchLib/Parallel RLC Branch  LConnTagsString=a  RConnTagsString=__new0  BranchType=RC  Resistance=0.5814618  Inductance=1e-3  SetiL0=off  InitialCurrent=0  Capacitance=0.01821425/0.5814618  Setx0=off  InitialVoltage=0  Measurements=None
  Voltage Measurement : spsVoltageMeasurementLib/Voltage Measurement  PhasorSimulation=off  OutputType=Complex  PSBequivalent=0
  Tj : Outport
  wires:
  Mean2/1 -> Tj/1
  [ambT] -> Controlled Voltage Source/1
  Ambient T/1 -> [ambT]
  Diode Power Loss/1 -> Controlled Current Source1/1
  Voltage Measurement/1 -> Mean2/1
  IGBT Power Loss/1 -> Controlled Current Source/1
  connections:
  Parallel RLC Branch5/RConn1 -- Parallel RLC Branch6/LConn1
  Parallel RLC Branch7/LConn1 -- Controlled Current Source1/RConn1
  Parallel RLC Branch7/RConn1 -- Parallel RLC Branch8/LConn1
  Parallel RLC Branch8/RConn1 -- Parallel RLC Branch9/LConn1
  Parallel RLC Branch9/RConn1 -- Parallel RLC Branch10/LConn1
  Controlled Current Source/RConn1 -- Voltage Measurement/LConn1 -- Parallel RLC Branch/LConn1
  Controlled Voltage Source/LConn1 -- Voltage Measurement/LConn2 -- Ground/LConn1
  Parallel RLC Branch6/RConn1 -- Controlled Current Source/LConn1 -- Controlled Current Source1/LConn1 -- Controlled Voltage Source/RConn1
  Parallel RLC Branch5/LConn1 -- Parallel RLC Branch10/RConn1 -- Parallel RLC Branch4/RConn1
  Parallel RLC Branch3/RConn1 -- Parallel RLC Branch4/LConn1
  Parallel RLC Branch2/RConn1 -- Parallel RLC Branch3/LConn1
  Parallel RLC Branch1/RConn1 -- Parallel RLC Branch2/LConn1
  Parallel RLC Branch/RConn1 -- Parallel RLC Branch1/LConn1

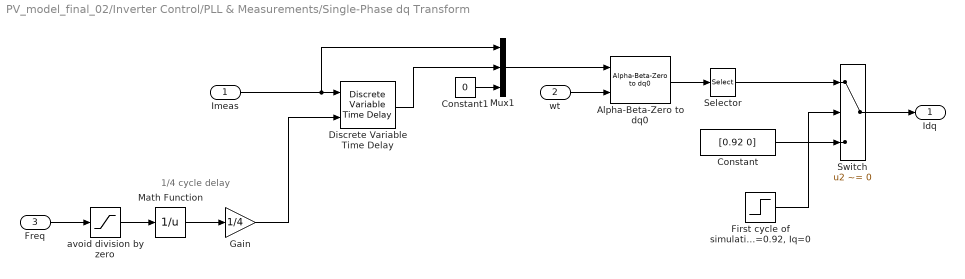
== system PV_model_final_02/Inverter Control/PLL & Measurements/Single-Phase dq Transform ==
  note: 1/4 cycle delay
  Imeas : Inport
  wt : Inport  Port=2
  Freq : Inport  Port=3
  Alpha-Beta-Zero to dq0 : spsAlphaBetaZerotodq0Lib/Alpha-Beta-Zero to dq0  Alignment=90 degrees behind phase A axis
      settings: SourceProductBaseCode=PS
  Constant : Constant  Value=[0.92 0]
  Constant1 : Constant  Value=0
  Discrete Variable Time Delay : spsDiscreteVariableTimeDelayLib/Discrete Variable Time Delay  MaxDelay=1  InitialValue=0  Ts=Ts_Control  DFT=on
      settings: SourceProductBaseCode=PS
  "First cycle of simulation Id=0.92, Iq=0" : Step  Time=1/Fnom  SampleTime=Ts_Control
  Gain : Gain  Gain=1/4
  Math Function : Math  Operator=reciprocal  SignedPower=on  SaturateOnIntegerOverflow=on
  Mux1 : Mux  Inputs=3
  Selector : Selector  InputPortWidth=3  IndexOptions=Index vector (dialog)  Indices=[1 2]  OutputSizes=1
  Switch : Switch  Criteria=u2 ~= 0
  avoid division by zero : Saturate  UpperLimit=60  LowerLimit=30
  Idq : Outport  VectorParamsAs1DForOutWhenUnconnected=off
  wires:
  Constant1/1 -> Mux1/3
  Discrete Variable Time Delay/1 -> Mux1/2
  Mux1/1 -> Alpha-Beta-Zero to dq0/1
  Imeas/1 -> Discrete Variable Time Delay/1, Mux1/1
  wt/1 -> Alpha-Beta-Zero to dq0/2
  Alpha-Beta-Zero to dq0/1 -> Selector/1
  Freq/1 -> avoid division by zero/1
  avoid division by zero/1 -> Math Function/1
  Math Function/1 -> Gain/1
  Gain/1 -> Discrete Variable Time Delay/2
  Selector/1 -> Switch/1
  Switch/1 -> Idq/1
  Constant/1 -> Switch/3
  "First cycle of simulation Id=0.92, Iq=0"/1 -> Switch/2

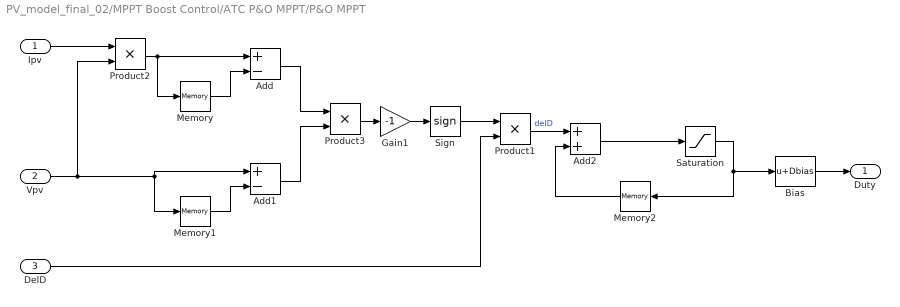
== system PV_model_final_02/MPPT Boost Control/ATC P&O MPPT/P&O MPPT ==
  Ipv : Inport
  Vpv : Inport  Port=2
  DelD : Inport  Port=3
  Add : Sum  Inputs=+-
  Add1 : Sum  Inputs=+-
  Add2 : Sum
  Bias : Bias  Bias=Dbias
  Gain1 : Gain  Gain=-1
  Memory : Memory
  Memory1 : Memory
  Memory2 : Memory
  Product1 : Product
  Product2 : Product
  Product3 : Product
  Saturation : Saturate  UpperLimit=Dupperlim  LowerLimit=Dlowerlim
  Sign : Signum
  Duty : Outport
  wires:
  Product3/1 -> Gain1/1
  Product1/1 -> Add2/1  "delD"
  Ipv/1 -> Product2/1
  Sign/1 -> Product1/1
  Add/1 -> Product3/1
  Memory1/1 -> Add1/2
  Memory2/1 -> Add2/2
  Memory/1 -> Add/2
  Product2/1 -> Memory/1, Add/1
  Add1/1 -> Product3/2
  Gain1/1 -> Sign/1
  DelD/1 -> Product1/2
  Vpv/1 -> Add1/1, Memory1/1, Product2/2
  Saturation/1 -> Bias/1, Memory2/1
  Add2/1 -> Saturation/1
  Bias/1 -> Duty/1
